simulink model "pwm"  (R2021b)
settings: Solver=VariableStepAuto  StartTime=0.0  StopTime=0.5  RelTol=1e-3
libraries: dspstat3 x1, simulink x1
settings Model: Creator=cirie  LastModifiedBy=cirie

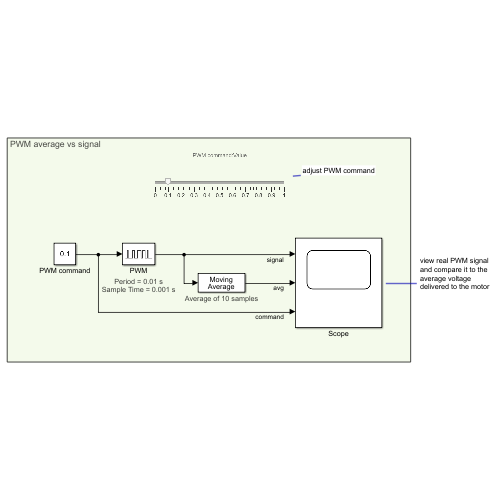
[thumbnail: Simulink's stored preview of the top-level diagram]
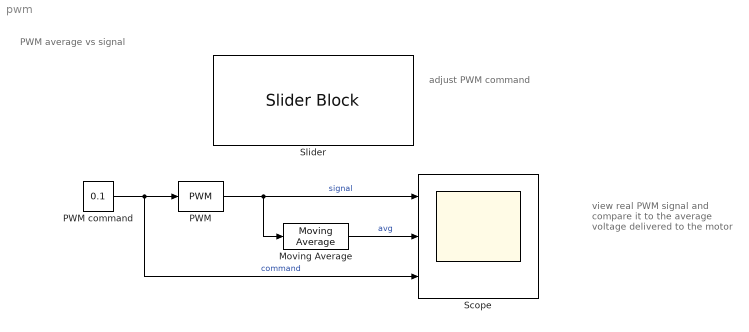
== system pwm ==
  note: adjust PWM command
  note: PWM average vs signal
  note: view real PWM signal and compare it to the average voltage delivered to the motor
  Moving Average : dspstat3/Moving Average  Method=Sliding window  ForgettingFactorPort=off  SpecifyWindowLength=on  WindowLength=10  ForgettingFactor=0.9  SimulateUsing=Interpreted execution
      settings: AttributesFormatString=Average of %<WindowLength> samples
  PWM : simulink/Discontinuities/PWM  DisableCoverage=on  Period=0.01  DisallowZeroDutyCycle=off  RunAtFixedTimeIntervals=on  SampleTime=0.001
      settings: AttributesFormatString=|
      | Period = %<Period> s
      | Sample Time = %<SampleTime> s
  PWM command : Constant  Value=0.1
  Scope : Scope  NumInputPorts=3
  Slider : SliderBlock  ScaleMax=1  TickInterval=0.1
  wires:
  PWM command/1 -> PWM/1, Scope/3  "command"
  PWM/1 -> Scope/1, Moving Average/1  "signal"
  Moving Average/1 -> Scope/2  "avg"
